simulink library "pathFollowingController_cl"  (R2018b)
settings: Solver=VariableStepAuto  StartTime=0.0  StopTime=10.0  RelTol=1e-3
undefined symbols (not defined in the file): env, FLIGHTCONTROLLER, fltCtrl, guess, initializeBussesFromBlock, kd_iter, ki_iter, kp_iter, Ten, vhcl
libraries: courseFollow_cl x1, ctrlAllocMatrix_cl x1, setpointToOutput_cl x1, spoolingController_cl x1
settings Model: Creator=jldanie5  LastModifiedBy=jldanie5

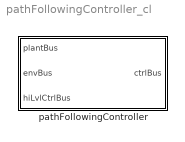
== system pathFollowingController_cl ==
  pathFollowingController : Subsystem  LoadFcn=initializeBussesFromBlock(gcb)  InitFcn=initializeBussesFromBlock(gcb)  StartFcn=initializeBussesFromBlock(gcb)  VariantControl=strcmpi(FLIGHTCONTROLLER,'pathFollowingController')  mask{initPosForInitSStar=vhcl.initPosVecGnd.Value, fluidDensity=env.water.density.Value, pathCtrl=fltCtrl, aeroStruct=vhcl.struct('OCT.aeroSurf')}
      mask prompts: initPosForInitSStar "Initial Position"; fluidDensity "Fluid Density"; pathCtrl "Controller"; aeroStruct "Aerodynamic Structure"
      mask DialogControl Container3 Prompt: courseFollow Params
      mask DialogControl Container4 Prompt: setpointToOutput Params

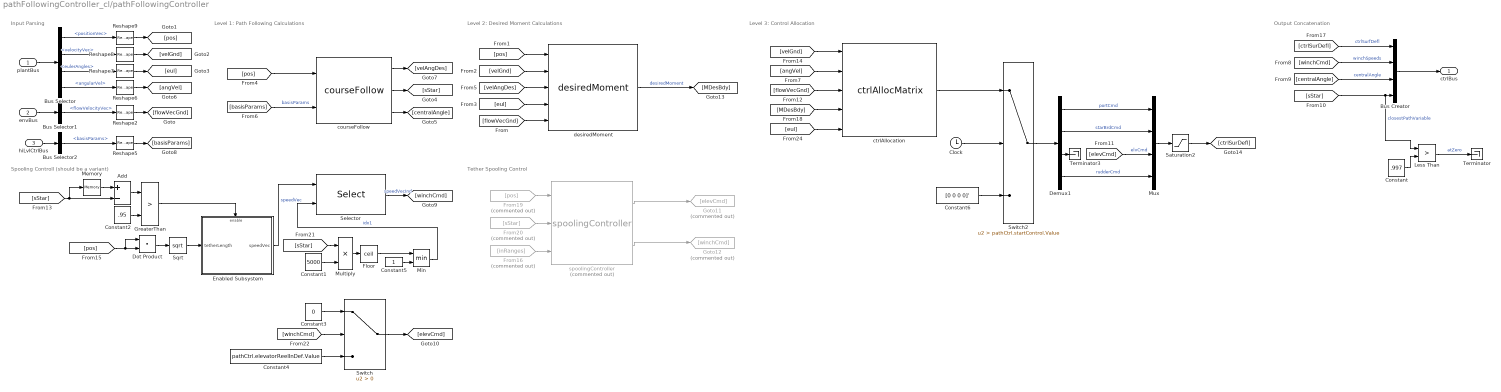
== system pathFollowingController_cl/pathFollowingController ==
  note: Level 3: Control Allocation
  note: Output Concatenation
  note: Tether Spooling Control
  note: Level 2: Desired Moment Calculations
  note: Level 1: Path Following Calculations
  note: Input Parsing
  note: Spooling Controll (should be a variant)
  plantBus : Inport  OutDataTypeStr=Bus: plantBus
  envBus : Inport  Port=2  OutDataTypeStr=Bus: envBus
  hiLvlCtrlBus : Inport  Port=3  OutDataTypeStr=Bus: hiLvlCtrlBus
  Add : Sum  Inputs=+-
  Bus Creator : BusCreator  Inputs=4  OutDataTypeStr=Bus: fltCtrlBus
      settings: InheritFromInputs=off
  Bus Selector : BusSelector  OutputSignals=positionVec,velocityVec,eulerAngles,angularVel
  Bus Selector1 : BusSelector  OutputSignals=flowVelocityVec
  Bus Selector2 : BusSelector  OutputSignals=basisParams
  Clock : Clock
  Constant : Constant  Value=.997
  Constant1 : Constant  Value=5000
  Constant2 : Constant  Value=.95
  Constant3 : Constant  Value=0
  Constant4 : Constant  Value=pathCtrl.elevatorReelInDef.Value
  Constant5 : Constant
  Constant6 : Constant  Value=[0 0 0 0]'
  Demux1 : Demux
  Dot Product : DotProduct  InputSameDT=on  OutDataTypeStr=Inherit: Inherit via internal rule
  Enabled Subsystem : Subsystem  TreatAsAtomicUnit=on
  Floor : Rounding  Operator=ceil
  From16 : From  Commented=on  GotoTag=inRanges
  From19 : From  Commented=on  GotoTag=pos
  From20 : From  Commented=on  GotoTag=sStar
  Goto11 : Goto  Commented=on  GotoTag=elevCmd
  Goto12 : Goto  Commented=on  GotoTag=winchCmd
  GreaterThan : RelationalOperator  Operator=>  OutDataTypeStr=boolean  RndMeth=Simplest
  Less Than : RelationalOperator  Operator=>  OutDataTypeStr=boolean  RndMeth=Simplest
  Memory : Memory  InitialCondition=pathCtrl.initPathVar.Value
  Min : MinMax  Inputs=2
  Multiply : Product
  Mux : Mux
  Reshape{2,5..9} (6 alike) : Reshape  OutputDimensionality=Column vector (2-D)
  Saturation2 : Saturate  UpperLimit=pathCtrl.controlSigMax.upperLimit.Value  LowerLimit=pathCtrl.controlSigMax.lowerLimit.Value
  Selector : Selector  InputPortWidth=5000  IndexOptions=Index vector (port)  Indices=[1 3]  OutputSizes=1
  Sqrt : Sqrt  SaturateOnIntegerOverflow=on
  Switch : Switch  Criteria=u2 > Threshold
  Switch2 : Switch  Criteria=u2 > Threshold  Threshold=pathCtrl.startControl.Value
  Terminator : Terminator
  Terminator3 : Terminator
  courseFollow : courseFollow_cl/courseFollow  SystemSampleTime=-1
  ctrlAllocation : ctrlAllocMatrix_cl/ctrlAllocMatrix  aeroStruct=aeroStruct  fluidDensity=fluidDensity  ctrlUpMax=pathCtrl.controlSigMax.upperLimit.Value  ctrlDnMax=pathCtrl.controlSigMax.lowerLimit.Value
  desiredMoment : setpointToOutput_cl/desiredMoment  SystemSampleTime=-1
  spoolingController : spoolingController_cl/spoolingController  Commented=on  SystemSampleTime=-1
  ctrlBus : Outport  OutDataTypeStr=Bus: fltCtrlBus
  wires:
  courseFollow/1 -> [velAngDes]
  plantBus/1 -> Bus Selector/1
  Bus Selector/2 -> Reshape8/1  "<velocityVec>"
  Bus Selector/1 -> Reshape9/1  "<positionVec>"
  Bus Selector/3 -> Reshape7/1  "<eulerAngles>"
  [pos] -> desiredMoment/1
  [velGnd] -> desiredMoment/2
  [eul] -> desiredMoment/4
  [pos] -> courseFollow/1
  Bus Creator/1 -> ctrlBus/1
  envBus/1 -> Bus Selector1/1
  Bus Selector1/1 -> Reshape2/1  "<flowVelocityVec>"
  [flowVecGnd] -> desiredMoment/5
  [winchCmd] -> Bus Creator/2  "winchSpeeds"
  courseFollow/2 -> [sStar]
  hiLvlCtrlBus/1 -> Bus Selector2/1
  [centralAngle] -> Bus Creator/3  "centralAngle"
  [sStar] -> Less Than/1, Bus Creator/4  "closestPathVariable"
  courseFollow/3 -> [centralAngle]
  desiredMoment/1 -> [MDesBdy]  "desiredMoment"
  Bus Selector/4 -> Reshape6/1  "<angularVel>"
  [angVel] -> ctrlAllocation/2
  [velGnd] -> ctrlAllocation/1
  [flowVecGnd] -> ctrlAllocation/3
  [elevCmd] -> Mux/3  "elvCmd"
  Mux/1 -> Saturation2/1
  Demux1/3 -> Terminator3/1
  Demux1/4 -> Mux/4  "rudderCmd"
  Demux1/1 -> Mux/1  "portCmd"
  Demux1/2 -> Mux/2  "starBrdCmd"
  [basisParams] -> courseFollow/2  "basisParams"
  Clock/1 -> Switch2/2
  Switch2/1 -> Demux1/1
  Constant6/1 -> Switch2/3
  spoolingController/1 -> Goto11/1
  spoolingController/2 -> Goto12/1
  From19/1 -> spoolingController/1
  From20/1 -> spoolingController/2
  [MDesBdy] -> ctrlAllocation/4
  ctrlAllocation/1 -> Switch2/1
  [ctrlSurDefl] -> Bus Creator/1  "ctrlSurfDefl"
  [velAngDes] -> desiredMoment/3
  Bus Selector2/1 -> Reshape5/1  "<basisParams>"
  Reshape5/1 -> [basisParams]
  Saturation2/1 -> [ctrlSurDefl]
  Reshape2/1 -> [flowVecGnd]
  Reshape6/1 -> [angVel]
  Reshape7/1 -> [eul]
  Reshape8/1 -> [velGnd]
  Reshape9/1 -> [pos]
  [eul] -> ctrlAllocation/5
  [sStar] -> Add/2, Memory/1
  Memory/1 -> Add/1
  Add/1 -> GreaterThan/1
  Constant2/1 -> GreaterThan/2
  GreaterThan/1 -> Enabled Subsystem/Enable
  [pos] -> Dot Product/1, Dot Product/2
  Dot Product/1 -> Sqrt/1
  Sqrt/1 -> Enabled Subsystem/1(tetherLength)
  From16/1 -> spoolingController/3
  Constant/1 -> Less Than/2
  Less Than/1 -> Terminator/1  "atZero"
  Selector/1 -> [winchCmd]  "speedVecInd"
  [sStar] -> Multiply/1
  Constant1/1 -> Multiply/2
  Multiply/1 -> Floor/1
  Enabled Subsystem/1(speedVec) -> Selector/1  "speedVec"
  [winchCmd] -> Switch/2
  Constant3/1 -> Switch/1
  Constant4/1 -> Switch/3
  Switch/1 -> [elevCmd]
  Floor/1 -> Min/1
  Constant5/1 -> Min/2
  Min/1 -> Selector/2  "idx1"

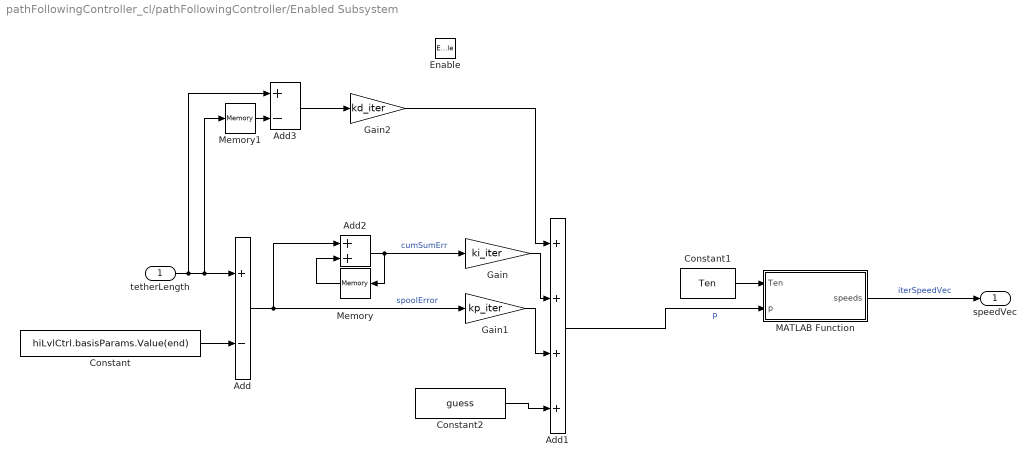
== system pathFollowingController_cl/pathFollowingController/Enabled Subsystem ==
  tetherLength : Inport
  Enable : EnablePort
  Add : Sum  Inputs=+-
  Add1 : Sum  Inputs=++++
  Add2 : Sum
  Add3 : Sum  Inputs=+-
  Constant : Constant  Value=hiLvlCtrl.basisParams.Value(end)
  Constant1 : Constant  Value=Ten
  Constant2 : Constant  Value=guess
  Gain : Gain  Gain=ki_iter
  Gain1 : Gain  Gain=kp_iter
  Gain2 : Gain  Gain=kd_iter
  MATLAB Function : MATLAB Function  TreatAsAtomicUnit=on
  Memory : Memory
  Memory1 : Memory
  speedVec : Outport
  wires:
  Add/1 -> Add2/1, Gain1/1  "spoolError"
  Add2/1 -> Memory/1, Gain/1  "cumSumErr"
  Gain/1 -> Add1/2
  Gain1/1 -> Add1/3
  MATLAB Function/1(speeds) -> speedVec/1  "iterSpeedVec"
  Add1/1 -> MATLAB Function/2(p)  "p"
  Constant1/1 -> MATLAB Function/1(Ten)
  Memory/1 -> Add2/2
  Constant2/1 -> Add1/4
  tetherLength/1 -> Add3/1, Memory1/1, Add/1
  Constant/1 -> Add/2
  Memory1/1 -> Add3/2
  Add3/1 -> Gain2/1
  Gain2/1 -> Add1/1

== matlab function pathFollowingController_cl/pathFollowingController/Enabled Subsystem/MATLAB Function ==
  data: Ten input; speeds output; p input
function speeds = fcn(Ten, p)
xopts=linspace(-.4,.4,1000);
speeds = zeros(1000,1);
for ii = 1:1000
    hamil = @(x) (p-Ten(ii,xopts==x)).*x;
    [~,bestind]=min(hamil(xopts));
    speeds(ii)=xopts(bestind);
end
